simulink model "ifelse"  (R2019b)
settings: Solver=VariableStepAuto  StartTime=0.0  StopTime=10.0  RelTol=1e-3
settings Model: Creator=omiks  LastModifiedBy=omiks

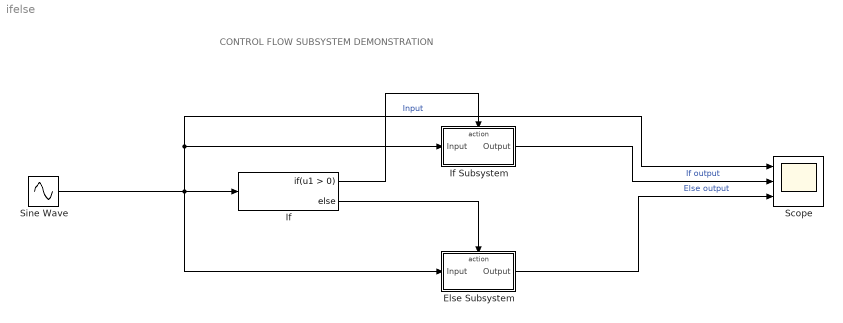
== system ifelse ==
  note: CONTROL FLOW SUBSYSTEM DEMONSTRATION
  Else Subsystem : Subsystem  TreatAsAtomicUnit=on
  "If " : If
  "If Subsystem " : Subsystem  TreatAsAtomicUnit=on
  Scope : Scope  NumInputPorts=3
  "Sine Wave " : Sin  SineType=Sample based  Frequency=5  Samples=2000  SampleTime=1/2000
  wires:
  "Sine Wave "/1 -> Scope/1, "If Subsystem "/1("Input "), Else Subsystem/1("Input "), "If "/1  "Input"
  "If "/1 -> "If Subsystem "/Action
  "If "/2 -> Else Subsystem/Action
  "If Subsystem "/1(Output) -> Scope/2  "If output"
  Else Subsystem/1(Output) -> Scope/3  "Else output"

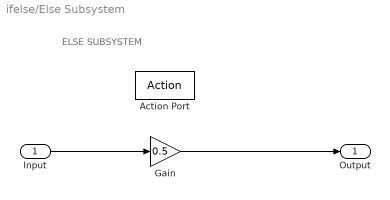
== system ifelse/Else Subsystem ==
  note: ELSE SUBSYSTEM
  "Input " : Inport
  Action Port : ActionPort  ActionPortLabel=else
  Gain : Gain  Gain=0.5
  Output : Outport
  wires:
  Gain/1 -> Output/1
  "Input "/1 -> Gain/1

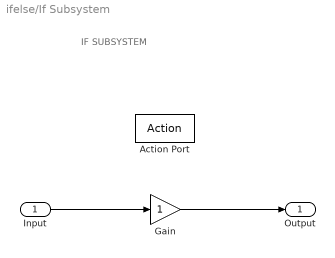
== system ifelse/If Subsystem  ==
  note: IF SUBSYSTEM
  "Input " : Inport
  Action Port : ActionPort  ActionPortLabel=if(u1 > 0)
  Gain : Gain
  Output : Outport
  wires:
  Gain/1 -> Output/1
  "Input "/1 -> Gain/1
